simulink model "UUV_ss_refinput"  (Simulink 8.0)
settings: Solver=ode45  StartTime=0.0  StopTime=10  RelTol=1e-3
values from neighbouring files (symbols this model uses):
  P =     [matlab.mat]
undefined symbols (not defined in the file or in its folder): controller_ref_input, drawUUV
libraries: simulink x1
settings Model: Creator=beard  LastModifiedBy=tmclain
settings DataIOCC: SignalLoggingSaveFormat=ModelDataLogs
settings OptimizationCC: InitFltsAndDblsToZero=on
settings DebuggingCC: FcnCallInpInsideContextMsg=UseLocalSettings  StrictBusMsg=Warning
settings GRTTargetCC: CombineOutputUpdateFcns=off  GRTInterface=on

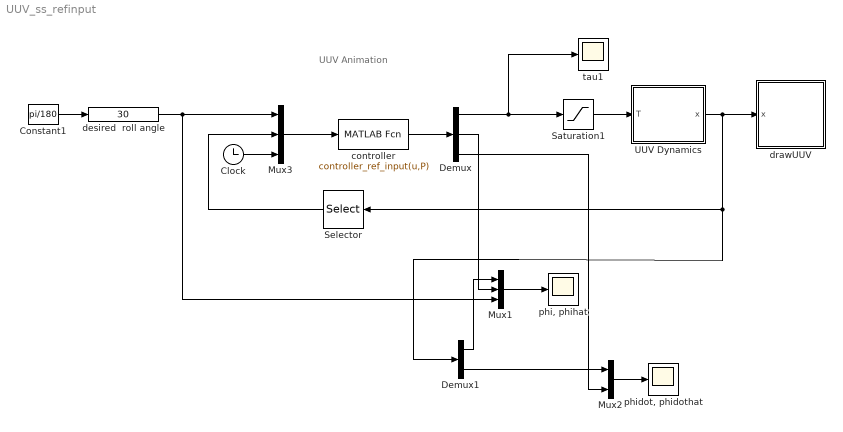
== system UUV_ss_refinput ==
  note: UUV Animation
  Clock : Clock
  Constant1 : Constant  Value=pi/180
  Demux : Demux  Outputs=3
  Demux1 : Demux  Outputs=2
  Mux1 : Mux  Inputs=3
  Mux2 : Mux  Inputs=2
  Mux3 : Mux  Inputs=3
  Saturation1 : Saturate  UpperLimit=250  LowerLimit=-250
  Selector : Selector  InputPortWidth=2  IndexOptions=Index vector (dialog)  Indices=[1]  OutputSizes=1
  UUV Dynamics : Subsystem
  controller : MATLABFcn  MATLABFcn=controller_ref_input(u,P)  OutputDimensions=3  SampleTime=P.Ts
  desired  roll angle : simulink/Math Operations/Slider Gain  low=-100  gain=30  high=100
  drawUUV : Subsystem
      mask init:
      | % drawing parameters
      | MajorAxis = 10;
      | MinorAxis = 6;
      | C_M = [0;-4];
      mask Display: image(imread('tv.jpg'))
  "phi, phihat" : Scope
      settings: TimeRange=10  YMin=0  YMax=0.7000000000000001  SaveName=ScopeData2
  "phidot, phidothat" : Scope
      settings: TimeRange=10  YMin=-0.1  YMax=0.6000000000000001  SaveName=ScopeData4
  tau1 : Scope
      settings: TimeRange=10  YMin=0  YMax=80  SaveName=ScopeData3
  wires:
  UUV Dynamics/1(x) -> drawUUV/1(x), Selector/1, Demux1/1
  Saturation1/1 -> UUV Dynamics/1(T)
  controller/1 -> Demux/1
  Demux/1 -> Saturation1/1, tau1/1
  Mux1/1 -> "phi, phihat"/1
  Demux1/1 -> Mux1/1
  Demux/2 -> Mux1/2
  Demux1/2 -> Mux2/1
  Demux/3 -> Mux2/2
  Mux2/1 -> "phidot, phidothat"/1
  Mux3/1 -> controller/1
  Clock/1 -> Mux3/3
  Selector/1 -> Mux3/2
  Constant1/1 -> desired  roll angle/1
  desired  roll angle/1 -> Mux1/3, Mux3/1

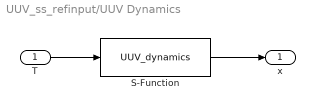
== system UUV_ss_refinput/UUV Dynamics ==
  T : Inport
  S-Function : S-Function  FunctionName=UUV_dynamics  Parameters=P  EnableBusSupport=off
  x : Outport
  wires:
  T/1 -> S-Function/1
  S-Function/1 -> x/1

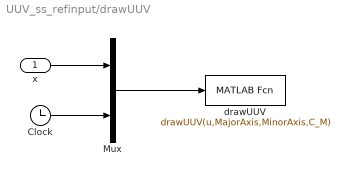
== system UUV_ss_refinput/drawUUV ==
  x : Inport
  Clock : Clock
  Mux : Mux  Inputs=2
  drawUUV : MATLABFcn  MATLABFcn=drawUUV(u,MajorAxis,MinorAxis,C_M)  OutputDimensions=0  SampleTime=0.1
  wires:
  Mux/1 -> drawUUV/1
  x/1 -> Mux/1
  Clock/1 -> Mux/2
